simulink model "AGTF30SysDyn_PExPIn"  (R2023b)
settings: Solver=ode4  StartTime=0.0  StopTime=MWS.In.tend  FixedStep=MWS.In.Ts  RelTol=1e-3  EnableMultiTasking=on
model workspace: external: MAT-File (data not in the file)
values from neighbouring files (symbols this model uses):
  MWS = setup_initialize(MWS,startPt,SSsolverSP)    [Setup_Simulation.m]    (also in run_AGTF30e_script.m = Setup_Simulation(inputMethod,MWS.In,filename,Mdl,SSsolverSP))
undefined symbols (not defined in the file or in its folder): DiscIntNeverNeededParam
libraries: simulink x32, Lib_Solve_ModelSource_TMATS x28, Lib_EMTAT x27, Lib_Cntrl_FirstOrderSensor_TMATS x19, Lib_Cntrl_FirstOrderActuator_TMATS x2, Lib_Cntrl_LimitSelect_TMATS x2, Lib_Solve_OuterLoopIntegrator_TMATS x2, Lib_Cntrl_CorrectedSpeed_TMATS x1, Lib_Solve_IterNRSolverJC_TMATS x1, slpidlib x1
(part 6 of 8)

== system AGTF30SysDyn_PExPIn/Control System/Scheduling/Steady State EM Power - MaxMin/HP and LP Pwr Calc/Gearbox Speeds/Spool to PGB speeds ==
  note: Sun
      | Ring
      | Carrier
  note: Sun
      | Ring
      | Carrier
  N : Inport
  Constant : Constant  Value=MWS.In.Options.PGBConfig
  Demux1 : Demux  Outputs=2
  Epicyclic Gearbox Speed Calc - RC : Subsystem  mask(Epicyclic Gearbox Speed Calc - SC){rS_M=MWS.Shaft.PGB.Sun.r, rR_M=MWS.Shaft.PGB.Ring.r}
      mask prompts: rS_M "rS_M - Sun gear radius, ft"; rR_M "rR_M - Ring gear radius, ft"
      mask help: This block outputs the rotational speeds of all 4 epicyclic gearbox components (sun, ring, carrier, planets) given the speeds of the sun gear and carrier. Units are consistent with input units.
      mask init:
      | rP_I = 0.5*(rR_M-rS_M);
  Epicyclic Gearbox Speed Calc - RC1 : Subsystem  mask(Epicyclic Gearbox Speed Calc - SC){rS_M=MWS.Shaft.PGB.Sun.r, rR_M=MWS.Shaft.PGB.Ring.r}
      mask prompts: rS_M "rS_M - Sun gear radius, ft"; rR_M "rR_M - Ring gear radius, ft"
      mask help: This block outputs the rotational speeds of all 4 epicyclic gearbox components (sun, ring, carrier, planets) given the speeds of the sun gear and carrier. Units are consistent with input units.
      mask init:
      | rP_I = 0.5*(rR_M-rS_M);
  Epicyclic Gearbox Speed Calc - SC : Subsystem  mask(Epicyclic Gearbox Speed Calc - SC){rS_M=MWS.Shaft.PGB.Sun.r, rR_M=MWS.Shaft.PGB.Ring.r}
      mask prompts: rS_M "rS_M - Sun gear radius, ft"; rR_M "rR_M - Ring gear radius, ft"
      mask help: This block outputs the rotational speeds of all 4 epicyclic gearbox components (sun, ring, carrier, planets) given the speeds of the sun gear and carrier. Units are consistent with input units.
      mask init:
      | rP_I = 0.5*(rR_M-rS_M);
  Epicyclic Gearbox Speed Calc - SC1 : Subsystem  mask(Epicyclic Gearbox Speed Calc - SC){rS_M=MWS.Shaft.PGB.Sun.r, rR_M=MWS.Shaft.PGB.Ring.r}
      mask prompts: rS_M "rS_M - Sun gear radius, ft"; rR_M "rR_M - Ring gear radius, ft"
      mask help: This block outputs the rotational speeds of all 4 epicyclic gearbox components (sun, ring, carrier, planets) given the speeds of the sun gear and carrier. Units are consistent with input units.
      mask init:
      | rP_I = 0.5*(rR_M-rS_M);
  Epicyclic Gearbox Speed Calc - SR : Subsystem  mask(Epicyclic Gearbox Speed Calc - SR){rS_M=MWS.Shaft.PGB.Sun.r, rR_M=MWS.Shaft.PGB.Ring.r}
      mask prompts: rS_M "rS_M - Radius of the sun gear, ft"; rR_M "rR_M - Radius of the ring gear, ft"
      mask help: This block outputs the rotational speeds of all 4 epicyclic gearbox components (sun, ring, carrier, planets) given the speeds of the sun gear and ring gear. Units are consistent with input units.
      mask init:
      | rP_I = 0.5*(rR_M-rS_M);
  Epicyclic Gearbox Speed Calc - SR1 : Subsystem  mask(Epicyclic Gearbox Speed Calc - SR){rS_M=MWS.Shaft.PGB.Sun.r, rR_M=MWS.Shaft.PGB.Ring.r}
      mask prompts: rS_M "rS_M - Radius of the sun gear, ft"; rR_M "rR_M - Radius of the ring gear, ft"
      mask help: This block outputs the rotational speeds of all 4 epicyclic gearbox components (sun, ring, carrier, planets) given the speeds of the sun gear and ring gear. Units are consistent with input units.
      mask init:
      | rP_I = 0.5*(rR_M-rS_M);
  Gain1 : Gain  Gain=MWS.Shaft.PGB.Sun.GR_gb %GR = Ngb/Nint
  Gain19 : Gain  Gain=MWS.Shaft.PGB.Ring.GR_gb %GR = Ngb/Nint
  Gain2 : Gain  Gain=MWS.Shaft.PGB.Sun.GR_int %GR = Nint/Ncomp
  Gain20 : Gain  Gain=MWS.Shaft.PGB.Carrier.GR_int %GR = Nint/Ncomp
  Gain21 : Gain  Gain=MWS.Shaft.PGB.Carrier.GR_gb %GR = Ngb/Nint
  Gain22 : Gain  Gain=MWS.Shaft.PGB.Ring.GR_int %GR = Nint/Ncomp
  Gain23 : Gain  Gain=MWS.Shaft.PGB.Sun.GR_gb %GR = Ngb/Nint
  Gain24 : Gain  Gain=MWS.Shaft.PGB.Ring.GR_gb %GR = Ngb/Nint
  Gain25 : Gain  Gain=MWS.Shaft.PGB.Sun.GR_int %GR = Nint/Ncomp
  Gain26 : Gain  Gain=MWS.Shaft.PGB.Carrier.GR_int %GR = Nint/Ncomp
  Gain27 : Gain  Gain=MWS.Shaft.PGB.Carrier.GR_gb %GR = Ngb/Nint
  Gain28 : Gain  Gain=MWS.Shaft.PGB.Ring.GR_int %GR = Nint/Ncomp
  Multiport Switch2 : MultiPortSwitch  Inputs=6  SaturateOnIntegerOverflow=off  InputSameDT=off
  NPGB : Outport
  wires:
  Demux1/1 -> Gain20/1, Gain22/1, Gain2/1  "N2"
  Gain27/1 -> [NC_HP]
  Epicyclic Gearbox Speed Calc - RC1/1(N) -> Multiport Switch2/7
  Epicyclic Gearbox Speed Calc - SR1/1(N) -> Multiport Switch2/4
  Gain22/1 -> Gain19/1
  [NS_LP] -> Epicyclic Gearbox Speed Calc - SR1/1(NS)
  [NR_LP] -> Epicyclic Gearbox Speed Calc - RC1/1(NR)
  N/1 -> Demux1/1
  Gain20/1 -> Gain21/1
  Gain28/1 -> Gain24/1
  [NC_LP] -> Epicyclic Gearbox Speed Calc - SC/2(NC)
  Gain2/1 -> Gain1/1
  [NS_HP] -> Epicyclic Gearbox Speed Calc - SC/1(NS)
  Multiport Switch2/1 -> NPGB/1
  [NR_LP] -> Epicyclic Gearbox Speed Calc - SR/2(NR)
  Gain24/1 -> [NR_HP]
  [NR_HP] -> Epicyclic Gearbox Speed Calc - RC/1(NR)
  Demux1/2 -> Gain26/1, Gain28/1, Gain25/1  "N3"
  Gain26/1 -> Gain27/1
  Gain25/1 -> Gain23/1
  Gain1/1 -> [NS_LP]
  Epicyclic Gearbox Speed Calc - SC/1(N) -> Multiport Switch2/3
  [NS_HP] -> Epicyclic Gearbox Speed Calc - SR/1(NS)
  Gain19/1 -> [NR_LP]
  Gain21/1 -> [NC_LP]
  Gain23/1 -> [NS_HP]
  Epicyclic Gearbox Speed Calc - SR/1(N) -> Multiport Switch2/2
  [NC_HP] -> Epicyclic Gearbox Speed Calc - SC1/2(NC)
  [NC_HP] -> Epicyclic Gearbox Speed Calc - RC1/2(NC)
  [NS_LP] -> Epicyclic Gearbox Speed Calc - SC1/1(NS)
  Epicyclic Gearbox Speed Calc - RC/1(N) -> Multiport Switch2/5
  Constant/1 -> Multiport Switch2/1
  [NR_HP] -> Epicyclic Gearbox Speed Calc - SR1/2(NR)
  [NC_LP] -> Epicyclic Gearbox Speed Calc - RC/2(NC)
  Epicyclic Gearbox Speed Calc - SC1/1(N) -> Multiport Switch2/6

== system AGTF30SysDyn_PExPIn/EngineSystem/Power System/Electrical Power System/EM Variant Subsystem/Scalar DEM Subsystem/PCabqPEM Calc ==
  CablePwr : Inport
  EMPwr : Inport  Port=2
  Divide1 : Product  Inputs=*/
  Memory : Memory  InitialCondition=1
  Saturation : Saturate  UpperLimit=1/0.2  LowerLimit=0.2
  Switch : Switch  Criteria=u2 > Threshold  SaturateOnIntegerOverflow=off  InputSameDT=off
  W to hp2 : Gain  Gain=1/745.7
  Zero Check2 : Subsystem
  PCabqPEM : Outport
  wires:
  Memory/1 -> Switch/1
  W to hp2/1 -> Divide1/1
  Zero Check2/2(Check) -> Switch/2
  Saturation/1 -> PCabqPEM/1, Memory/1
  CablePwr/1 -> W to hp2/1
  Zero Check2/1(EMPwrNZ) -> Divide1/2
  EMPwr/1 -> Zero Check2/1(EMPwr)
  Divide1/1 -> Switch/3
  Switch/1 -> Saturation/1

== system AGTF30SysDyn_PExPIn/EngineSystem/Power System/Electrical Power System/EM Variant Subsystem/Scalar DEM Subsystem/PCabqPEM Calc1 ==
  CablePwr : Inport
  EMPwr : Inport  Port=2
  Divide1 : Product  Inputs=*/
  Memory : Memory  InitialCondition=1
  Saturation : Saturate  UpperLimit=1/0.2  LowerLimit=0.2
  Switch : Switch  Criteria=u2 > Threshold  SaturateOnIntegerOverflow=off  InputSameDT=off
  W to hp2 : Gain  Gain=1/745.7
  Zero Check2 : Subsystem
  PCabqPEM : Outport
  wires:
  Switch/1 -> Saturation/1
  Divide1/1 -> Switch/3
  EMPwr/1 -> Zero Check2/1(EMPwr)
  Zero Check2/1(EMPwrNZ) -> Divide1/2
  CablePwr/1 -> W to hp2/1
  Saturation/1 -> Memory/1, PCabqPEM/1
  Zero Check2/2(Check) -> Switch/2
  W to hp2/1 -> Divide1/1
  Memory/1 -> Switch/1

== system AGTF30SysDyn_PExPIn/EngineSystem/Power System/Electrical Power System/EM Variant Subsystem/Scalar PGB EM Subsystem/PCabqPEM Calc ==
  CablePwr : Inport
  EMPwr : Inport  Port=2
  Divide1 : Product  Inputs=*/
  Memory : Memory  InitialCondition=1
  Saturation : Saturate  UpperLimit=1/0.2  LowerLimit=0.2
  Switch : Switch  Criteria=u2 > Threshold  SaturateOnIntegerOverflow=off  InputSameDT=off
  W to hp2 : Gain  Gain=1/745.7
  Zero Check2 : Subsystem
  PCabqPEM : Outport
  wires:
  Memory/1 -> Switch/1
  W to hp2/1 -> Divide1/1
  Zero Check2/2(Check) -> Switch/2
  Saturation/1 -> PCabqPEM/1, Memory/1
  CablePwr/1 -> W to hp2/1
  Zero Check2/1(EMPwrNZ) -> Divide1/2
  EMPwr/1 -> Zero Check2/1(EMPwr)
  Switch/1 -> Saturation/1
  Divide1/1 -> Switch/3

== system AGTF30SysDyn_PExPIn/EngineSystem/Power System/Electrical Power System/EM Variant Subsystem/Scalar PGB EM Subsystem/PCabqPEM Calc1 ==
  CablePwr : Inport
  EMPwr : Inport  Port=2
  Divide1 : Product  Inputs=*/
  Memory : Memory  InitialCondition=1
  Saturation : Saturate  UpperLimit=1/0.2  LowerLimit=0.2
  Switch : Switch  Criteria=u2 > Threshold  SaturateOnIntegerOverflow=off  InputSameDT=off
  W to hp2 : Gain  Gain=1/745.7
  Zero Check2 : Subsystem
  PCabqPEM : Outport
  wires:
  Memory/1 -> Switch/1
  W to hp2/1 -> Divide1/1
  Zero Check2/2(Check) -> Switch/2
  Saturation/1 -> PCabqPEM/1, Memory/1
  CablePwr/1 -> W to hp2/1
  Zero Check2/1(EMPwrNZ) -> Divide1/2
  EMPwr/1 -> Zero Check2/1(EMPwr)
  Divide1/1 -> Switch/3
  Switch/1 -> Saturation/1

== system AGTF30SysDyn_PExPIn/EngineSystem/Power System/Electrical Power System/EM Variant Subsystem/Scalar PGB EM Subsystem/PCabqPEM Calc2 ==
  CablePwr : Inport
  EMPwr : Inport  Port=2
  Divide1 : Product  Inputs=*/
  Memory : Memory  InitialCondition=1
  Saturation : Saturate  UpperLimit=1/0.2  LowerLimit=0.2
  Switch : Switch  Criteria=u2 > Threshold  SaturateOnIntegerOverflow=off  InputSameDT=off
  W to hp2 : Gain  Gain=1/745.7
  Zero Check2 : Subsystem
  PCabqPEM : Outport
  wires:
  Memory/1 -> Switch/1
  W to hp2/1 -> Divide1/1
  Zero Check2/2(Check) -> Switch/2
  Saturation/1 -> PCabqPEM/1, Memory/1
  CablePwr/1 -> W to hp2/1
  Zero Check2/1(EMPwrNZ) -> Divide1/2
  EMPwr/1 -> Zero Check2/1(EMPwr)
  Divide1/1 -> Switch/3
  Switch/1 -> Saturation/1

== system AGTF30SysDyn_PExPIn/EngineSystem/Power System/Electrical Power System/EM Variant Subsystem/Scalar PGB EM Subsystem/PCabqPEM Calc3 ==
  CablePwr : Inport
  EMPwr : Inport  Port=2
  Divide1 : Product  Inputs=*/
  Memory : Memory  InitialCondition=1
  Saturation : Saturate  UpperLimit=1/0.2  LowerLimit=0.2
  Switch : Switch  Criteria=u2 > Threshold  SaturateOnIntegerOverflow=off  InputSameDT=off
  W to hp2 : Gain  Gain=1/745.7
  Zero Check2 : Subsystem
  PCabqPEM : Outport
  wires:
  Memory/1 -> Switch/1
  W to hp2/1 -> Divide1/1
  Zero Check2/2(Check) -> Switch/2
  Saturation/1 -> PCabqPEM/1, Memory/1
  CablePwr/1 -> W to hp2/1
  Zero Check2/1(EMPwrNZ) -> Divide1/2
  EMPwr/1 -> Zero Check2/1(EMPwr)
  Divide1/1 -> Switch/3
  Switch/1 -> Saturation/1

== system AGTF30SysDyn_PExPIn/EngineSystem/Power System/Electrical Power System/Energy Storage Subsystem/DCDC Variant Subsystem/DCDC Regulator Subsystem ==
  V_ESD [V] : Inport
  I_Bus [A] : Inport  Port=2
  Constant : Constant  Value=MWS.EPS.DCDC.Vset
  Constant129 : Constant  Value=0
  Constant39 : Constant  Value=0
  DC-DC Converter (Efficiency Map) (Regulate Output Voltage) : Lib_EMTAT/Components/Power Flow/DC-DC Converter (Efficiency Map) (Regulate Output Voltage)  X_Vin_VoltageVec_M=MWS.EPS.DCDC.Vvec  Y_Iout_CurrentVec_M=MWS.EPS.DCDC.Ivec  T_C_EffArray_M=MWS.EPS.DCDC.Eff  FM=0
      settings: SourceProductName=EMTAT
      settings: AttributesFormatString=|
      | DC-DC Converter
      | (Efficiency Map)
      | (Regulate Output Voltage)
  Electrical Bus : Lib_EMTAT/Components/Power Flow/Electrical Bus  C=MWS.EPS.Bus.C  Nb=1
      settings: AttributesFormatString=Electrical Bus  SourceProductName=EMTAT
  Gain : Gain  Gain=-1
  Gain1 : Gain  Gain=-1
  Integrator : Integrator  InitialCondition=MWS.EPS.Bus.Vout_IC
  Mux : Mux  Inputs=2
  PID Controller : slpidlib/PID Controller  Controller=PID  Form=Parallel  TimeDomain=Continuous-time  UseExternalTs=off  SampleTime=-1  IntegratorMethod=Forward Euler  FilterMethod=Forward Euler  ControllerParametersSource=internal  P=MWS.EPS.DCDC.PID.kp  I=MWS.EPS.DCDC.PID.ki  UseKiTs=off  D=MWS.EPS.DCDC.PID.kd  N=100  UseFilter=on  TunerSelectOption=Frequency Response Based  InitialConditionSource=internal  InitialConditionForIntegrator=0  InitialConditionForFilter=0  DifferentiatorICPrevScaledInput=0  ExternalReset=none  TrackingMode=off  Kt=1  LimitOutput=off  SatLimitsSource=internal  UpperSaturationLimit=inf  LowerSaturationLimit=-inf  LinearizeAsGain=on  AntiWindupMode=none  Kb=1  LimitIntegrator=off  UpperIntegratorSaturationLimit=inf  LowerIntegratorSaturationLimit=-inf  POutMin=[]  POutMax=[]  IOutMin=[]  IOutMax=[]  DOutMin=[]  DOutMax=[]  NOutMin=[]  NOutMax=[]  SumOutMin=[]  SumOutMax=[]  SaturationOutMin=[]  SaturationOutMax=[]  PParamMin=[]  PParamMax=[]  IParamMin=[]  IParamMax=[]  DParamMin=[]  DParamMax=[]  NParamMin=[]  NParamMax=[]  KbParamMin=[]  KbParamMax=[]  KtParamMin=[]  KtParamMax=[]  KbOutMin=[]  KbOutMax=[]  KtOutMin=[]  KtOutMax=[]  IntegratorOutMin=[]  IntegratorOutMax=[]  FilterOutMin=[]  FilterOutMax=[]  SumI1OutMin=[]  SumI1OutMax=[]  SumI2OutMin=[]  SumI2OutMax=[]  SumI3OutMin=[]  SumI3OutMax=[]  SumI4OutMin=[]  SumI4OutMax=[]  SumDOutMin=[]  SumDOutMax=[]  DifferentiatorOutMin=[]  DifferentiatorOutMax=[]  FilterDiffOutCoefMin=[]  FilterDiffOutCoefMax=[]  ReciprocalOutMin=[]  ReciprocalOutMax=[]  SumDenOutMin=[]  SumDenOutMax=[]  SumNumOutMin=[]  SumNumOutMax=[]  DivideOutMin=[]  DivideOutMax=[]  UdiffTsProdOutMin=[]  UdiffTsProdOutMax=[]  NTsProdOutMin=[]  NTsProdOutMax=[]  UintegralTsProdOutMin=[]  UintegralTsProdOutMax=[]  UngainTsProdOutMin=[]  UngainTsProdOutMax=[]  ClampingZeroOutDataTypeStr=Inherit: Inherit via back propagation  ClampingZeroOutMin=[]  ClampingZeroOutMax=[]  FilterDenConstantOutDataTypeStr=Inherit: Inherit via back propagation  FilterDenConstantOutMin=[]  FilterDenConstantOutMax=[]  PCopyOutDataTypeStr=Inherit: Inherit via back propagation  PCopyOutMin=[]  PCopyOutMax=[]  NCopyOutDataTypeStr=Inherit: Inherit via back propagation  NCopyOutMin=[]  NCopyOutMax=[]  IntegratorContinuousStateAttributes=''  IntegratorStateMustResolveToSignalObject=off  IntegratorRTWStateStorageClass=Auto  FilterContinuousStateAttributes=''  FilterStateMustResolveToSignalObject=off  FilterRTWStateStorageClass=Auto  ParallelPVariant=InternalParameters  IdealPVariant=Disabled  IVariant=InternalParameters  DVariant=InternalParameters  IntegratorVariant=Continuous  SatVariant=Disabled  AWVariant=Passthrough  PCopyVariant=Disabled  TRVariant=Disabled  FdbkBlocksVariant=Forward  IdealPFdbkVariant=Disabled  SatFdbkVariant=Disabled  DerivativeFilterVariant=ContFilter  NVariant=InternalParameters  NCopyVariant=Disabled  FilterICVariant=InternalICsFilter  IntegratorICVariant=InternalICs  ExternalResetVariant=Disabled  TRSumVariant=Passthrough  SumFdbkVariant=Disabled  SumVariant=Sum_PID  TsampFilterVariant=InternalTs  TsampNgainVariant=Passthrough  TsampIntegralVariant=Disabled_SignalSpec  ExternalSaturationOutDataTypeStr=Inherit: Same as second input
  Sum : Sum  Inputs=-+
  Sum of Elements : Sum  Inputs=+
  Terminator46 : Terminator
  Vo [V] : Outport
  Io [A] : Outport  Port=2
  Outputs : Outport  Port=3
  wires:
  Constant39/1 -> DC-DC Converter (Efficiency Map) (Regulate Output Voltage)/4
  I_Bus [A]/1 -> Mux/2
  Constant129/1 -> DC-DC Converter (Efficiency Map) (Regulate Output Voltage)/5
  DC-DC Converter (Efficiency Map) (Regulate Output Voltage)/2 -> Terminator46/1
  DC-DC Converter (Efficiency Map) (Regulate Output Voltage)/1 -> Outputs/1
  Electrical Bus/2 -> Integrator/1
  Integrator/1 -> Electrical Bus/2
  Electrical Bus/1 -> Vo [V]/1, DC-DC Converter (Efficiency Map) (Regulate Output Voltage)/2, Sum/1
  DC-DC Converter (Efficiency Map) (Regulate Output Voltage)/3 -> Gain/1
  Constant/1 -> Sum/2
  PID Controller/1 -> DC-DC Converter (Efficiency Map) (Regulate Output Voltage)/3
  Sum/1 -> PID Controller/1
  Gain/1 -> Mux/1
  Sum of Elements/1 -> Gain1/1
  Gain1/1 -> Electrical Bus/1
  V_ESD [V]/1 -> DC-DC Converter (Efficiency Map) (Regulate Output Voltage)/1
  DC-DC Converter (Efficiency Map) (Regulate Output Voltage)/4 -> Io [A]/1
  Mux/1 -> Sum of Elements/1

== system AGTF30SysDyn_PExPIn/EngineSystem/Power System/Electrical Power System/Energy Storage Subsystem/DCDC Variant Subsystem/DCDC Set Point Subsystem ==
  V_ESD [V] : Inport
  I_Bus [A] : Inport  Port=2
  Constant : Constant  Value=MWS.EPS.DCDC.Vset
  Constant129 : Constant  Value=0
  Constant39 : Constant  Value=0
  DC-DC Converter (Efficiency Map) (Regulate Output Voltage) : Lib_EMTAT/Components/Power Flow/DC-DC Converter (Efficiency Map) (Regulate Output Voltage)  X_Vin_VoltageVec_M=MWS.EPS.DCDC.Vvec  Y_Iout_CurrentVec_M=MWS.EPS.DCDC.Ivec  T_C_EffArray_M=MWS.EPS.DCDC.Eff  FM=0
      settings: SourceProductName=EMTAT
      settings: AttributesFormatString=|
      | DC-DC Converter
      | (Efficiency Map)
      | (Regulate Output Voltage)
  Terminator46 : Terminator
  Unit Delay1 : UnitDelay  SampleTime=-1  HasFrameUpgradeWarning=on
  Vo [V] : Outport
  Io [A] : Outport  Port=2
  Outputs : Outport  Port=3
  wires:
  Constant39/1 -> DC-DC Converter (Efficiency Map) (Regulate Output Voltage)/4
  DC-DC Converter (Efficiency Map) (Regulate Output Voltage)/2 -> Outputs/1
  Constant/1 -> DC-DC Converter (Efficiency Map) (Regulate Output Voltage)/1
  V_ESD [V]/1 -> DC-DC Converter (Efficiency Map) (Regulate Output Voltage)/2
  Constant129/1 -> DC-DC Converter (Efficiency Map) (Regulate Output Voltage)/5
  I_Bus [A]/1 -> DC-DC Converter (Efficiency Map) (Regulate Output Voltage)/3
  DC-DC Converter (Efficiency Map) (Regulate Output Voltage)/4 -> Unit Delay1/1
  DC-DC Converter (Efficiency Map) (Regulate Output Voltage)/3 -> Terminator46/1
  DC-DC Converter (Efficiency Map) (Regulate Output Voltage)/1 -> Vo [V]/1
  Unit Delay1/1 -> Io [A]/1

== system AGTF30SysDyn_PExPIn/EngineSystem/Power System/Electrical Power System/Energy Storage Subsystem/ESD Variant Subsystem/ESD Battery Subsystem ==
  I [A] : Inport
  Battery : Lib_EMTAT/Components/Power Flow/Battery  ESR=MWS.EPS.Batt.ESR  Vcharge_vec=MWS.EPS.Batt.VCC  Vdischarge_vec=MWS.EPS.Batt.VDC  It_vec=MWS.EPS.Batt.DoD
      settings: AttributesFormatString=Battery  SourceProductName=EMTAT
  Bus Selector : BusSelector  OutputSignals=SoC; %
  Integrator : Integrator  InitialCondition=MWS.EPS.Batt.DoD_IC
  Terminator46 : Terminator
  Vo [V] : Outport
  SoC [%] : Outport  Port=2
  wires:
  Bus Selector/1 -> SoC [%]/1  "<SoC; %>"
  Battery/2 -> Bus Selector/1
  I [A]/1 -> Battery/1
  Battery/4 -> Integrator/1
  Integrator/1 -> Battery/2
  Battery/3 -> Terminator46/1
  Battery/1 -> Vo [V]/1

== system AGTF30SysDyn_PExPIn/EngineSystem/Power System/Electrical Power System/Energy Storage Subsystem/ESD Variant Subsystem/ESD Supercapacitor Subsystem ==
  I [A] : Inport
  Bus Selector : BusSelector  OutputSignals=SOC; %
  Integrator : Integrator  InitialCondition=MWS.EPS.SC.Vout_IC
  Supercapacitor : Lib_EMTAT/Components/Power Flow/Supercapacitor  C=MWS.EPS.SC.C  ESR=MWS.EPS.SC.ESR  TSE=MWS.EPS.SC.TSE  BlkNm=double(gcb)
      settings: AttributesFormatString=Supercapacitor  SourceProductName=EMTAT
  Terminator46 : Terminator
  Unit Delay : UnitDelay  InitialCondition=MWS.EPS.SC.Iout_IC  SampleTime=-1  HasFrameUpgradeWarning=on
  Vo [V] : Outport
  SoC [%] : Outport  Port=2
  wires:
  Integrator/1 -> Supercapacitor/2
  Supercapacitor/4 -> Integrator/1
  Supercapacitor/3 -> Terminator46/1
  Supercapacitor/1 -> Vo [V]/1  "Vout (Supercapacitor) [V]"
  Supercapacitor/5 -> Unit Delay/1
  Unit Delay/1 -> Supercapacitor/3
  I [A]/1 -> Supercapacitor/1
  Supercapacitor/2 -> Bus Selector/1
  Bus Selector/1 -> SoC [%]/1  "<SOC; %>"

== system AGTF30SysDyn_PExPIn/Control System/Electric Machine Controllers/EM Controllers/PGB EM Control/VEATE EM Controllers/Base Power/Base Power - Boost and PEx ==
  note: 1: HP-Sun, LP-Ring, Coupling-Carrier
      | 2: HP-Sun, LP-Carrier, Coupling-Ring
      | 3: HP-Ring, LP-Sun, Coupling-Carrier
      | 4: HP-Ring, LP-Carrier, Coupling-Sun
      | 5: HP-Carrier, LP-Sun, Coupling-Ring
      | 6: HP-Carrier, LP-Ring, Coupling-Sun
  note: PLANETARY GEARBOX EFFECT ON POWER TRANSFER
  PwrL_Base : Inport
  PwrH_Base : Inport  Port=2
  NS : Inport  Port=3
  NR : Inport  Port=4
  NC : Inport  Port=5
  Boost PEx - HC LR CS : Subsystem
  Boost PEx - HC LS CR : Subsystem
  Boost PEx - HR LC CS : Subsystem
  Boost PEx - HR LS CC : Subsystem
  Boost PEx - HS LC CR : Subsystem
  Boost PEx - HS LR CC : Subsystem
  CTrqCR : Constant  Value=MWS.Shaft.PGB.TrqCoeff.CTrqCR
  CTrqCS : Constant  Value=MWS.Shaft.PGB.TrqCoeff.CTrqCS
  CTrqRC : Constant  Value=MWS.Shaft.PGB.TrqCoeff.CTrqRC
  CTrqRS : Constant  Value=MWS.Shaft.PGB.TrqCoeff.CTrqRS
  CTrqSC : Constant  Value=MWS.Shaft.PGB.TrqCoeff.CTrqSC
  CTrqSR : Constant  Value=MWS.Shaft.PGB.TrqCoeff.CTrqSR
  Constant1 : Constant  Value=MWS.In.Options.PGBConfig
  Constant2 : Constant  Value=MWS.In.Options.PGBConfig
  Constant3 : Constant  Value=MWS.In.Options.PGBConfig
  Divide{4..7,12..13} (6 alike) : Product  Inputs=**/
  Multiport Switch1 : MultiPortSwitch  Inputs=6  SaturateOnIntegerOverflow=off  InputSameDT=off
  Multiport Switch4 : MultiPortSwitch  Inputs=6  SaturateOnIntegerOverflow=off  InputSameDT=off
  Multiport Switch8 : MultiPortSwitch  Inputs=6  SaturateOnIntegerOverflow=off  InputSameDT=off
  Mux{1..6} (6 alike) : Mux
  Pem : Outport
  wires:
  Boost PEx - HC LS CR/1(PemS_Base) -> Mux5/1
  Boost PEx - HC LR CS/1(PemS_Base) -> Mux6/1
  Boost PEx - HC LS CR/4(PemP_Base) -> Mux5/4
  Boost PEx - HC LR CS/2(PemR_Base) -> Mux6/2
  Boost PEx - HC LR CS/3(PemC_Base) -> Mux6/3
  Mux4/1 -> [Pem_HRLCCS]
  Mux6/1 -> [Pem_HCLRCS]
  Boost PEx - HC LS CR/3(PemC_Base) -> Mux5/3
  Boost PEx - HS LC CR/3(PemC_Base) -> Mux2/3
  Boost PEx - HS LR CC/2(PemR_Base) -> Mux1/2
  Boost PEx - HR LS CC/1(PemS_Base) -> Mux3/1
  Mux1/1 -> [Pem_HSLRCC]
  Boost PEx - HS LR CC/4(PemP_Base) -> Mux1/4
  Constant1/1 -> Multiport Switch4/1
  [Pem_HSLCCR] -> Multiport Switch4/3
  Boost PEx - HC LR CS/4(PemP_Base) -> Mux6/4
  [Pem_HRLCCS] -> Multiport Switch4/5
  Boost PEx - HS LC CR/1(PemS_Base) -> Mux2/1
  Boost PEx - HC LS CR/2(PemR_Base) -> Mux5/2
  Boost PEx - HS LC CR/2(PemR_Base) -> Mux2/2
  Boost PEx - HS LC CR/4(PemP_Base) -> Mux2/4
  Boost PEx - HR LS CC/2(PemR_Base) -> Mux3/2
  Mux5/1 -> [Pem_HCLSCR]
  Boost PEx - HR LC CS/2(PemR_Base) -> Mux4/2
  Boost PEx - HR LS CC/4(PemP_Base) -> Mux3/4
  [Pem_HCLSCR] -> Multiport Switch4/6
  Boost PEx - HR LS CC/3(PemC_Base) -> Mux3/3
  Boost PEx - HR LC CS/3(PemC_Base) -> Mux4/3
  [Pem_HSLRCC] -> Multiport Switch4/2
  Mux3/1 -> [Pem_HRLSCC]
  Boost PEx - HR LC CS/4(PemP_Base) -> Mux4/4
  Boost PEx - HR LC CS/1(PemS_Base) -> Mux4/1
  Boost PEx - HS LR CC/3(PemC_Base) -> Mux1/3
  Boost PEx - HS LR CC/1(PemS_Base) -> Mux1/1
  [Pem_HCLRCS] -> Multiport Switch4/7
  [Pem_HRLSCC] -> Multiport Switch4/4
  Multiport Switch4/1 -> Pem/1
  Mux2/1 -> [Pem_HSLCCR]
  [K_PXeffRC] -> Multiport Switch8/4
  [K_PXeffCR] -> Multiport Switch8/6
  [K_PXeffSC] -> Multiport Switch8/2
  [K_PXeffCR] -> Multiport Switch1/3
  Multiport Switch1/1 -> [K_PXeffL]
  [K_PXeffCS] -> Multiport Switch1/5
  [K_PXeffSC] -> Multiport Switch1/4
  Constant3/1 -> Multiport Switch1/1
  [K_PXeffCS] -> Multiport Switch8/7
  CTrqRC/1 -> Divide12/1
  Divide7/1 -> [K_PXeffRS]
  [NC] -> Divide6/3
  [NS] -> Divide5/2
  [NS] -> Divide13/3
  Divide5/1 -> [K_PXeffSR]
  Divide12/1 -> [K_PXeffRC]
  CTrqSR/1 -> Divide5/1
  Multiport Switch8/1 -> [K_PXeffH]
  [NS] -> Divide6/2
  [NR] -> Divide7/2
  Divide13/1 -> [K_PXeffCS]
  [K_PXeffRS] -> Multiport Switch1/7
  CTrqCS/1 -> Divide13/1
  [NR] -> Divide5/3
  [K_PXeffRC] -> Multiport Switch1/2
  [NR] -> Divide12/2
  Constant2/1 -> Multiport Switch8/1
  [NR] -> Divide4/3
  CTrqCR/1 -> Divide4/1
  CTrqRS/1 -> Divide7/1
  [NC] -> Divide13/2
  CTrqSC/1 -> Divide6/1
  Divide6/1 -> [K_PXeffSC]
  [K_PXeffSR] -> Multiport Switch8/3
  Divide4/1 -> [K_PXeffCR]
  [NC] -> Divide4/2
  [NC] -> Divide12/3
  [K_PXeffSR] -> Multiport Switch1/6
  [NS] -> Divide7/3
  [K_PXeffRS] -> Multiport Switch8/5
  PwrL_Base/1 -> [PwrL_Base]
  PwrH_Base/1 -> [PwrH_Base]
  NS/1 -> [NS]
  NR/1 -> [NR]
  NC/1 -> [NC]
  [PwrH_Base] -> Boost PEx - HS LR CC/2(PwrH_Base), Boost PEx - HC LR CS/2(PwrH_Base), Boost PEx - HC LS CR/2(PwrH_Base), Boost PEx - HR LC CS/2(PwrH_Base), Boost PEx - HR LS CC/2(PwrH_Base), Boost PEx - HS LC CR/2(PwrH_Base)
  [PwrL_Base] -> Boost PEx - HS LR CC/1(PwrL_Base), Boost PEx - HC LR CS/1(PwrL_Base), Boost PEx - HC LS CR/1(PwrL_Base), Boost PEx - HR LC CS/1(PwrL_Base), Boost PEx - HR LS CC/1(PwrL_Base), Boost PEx - HS LC CR/1(PwrL_Base)
  [K_PXeffH] -> Boost PEx - HS LR CC/4(K_PXeffH), Boost PEx - HC LR CS/4(K_PXeffH), Boost PEx - HC LS CR/4(K_PXeffH), Boost PEx - HR LC CS/4(K_PXeffH), Boost PEx - HR LS CC/4(K_PXeffH), Boost PEx - HS LC CR/4(K_PXeffH)
  [K_PXeffL] -> Boost PEx - HS LR CC/3(K_PXeffL), Boost PEx - HC LR CS/3(K_PXeffL), Boost PEx - HC LS CR/3(K_PXeffL), Boost PEx - HR LC CS/3(K_PXeffL), Boost PEx - HR LS CC/3(K_PXeffL), Boost PEx - HS LC CR/3(K_PXeffL)
  [NS] -> Boost PEx - HS LR CC/5(NS), Boost PEx - HC LR CS/5(NS), Boost PEx - HC LS CR/5(NS), Boost PEx - HR LC CS/5(NS), Boost PEx - HR LS CC/5(NS), Boost PEx - HS LC CR/5(NS)
  [NR] -> Boost PEx - HS LR CC/6(NR), Boost PEx - HC LR CS/6(NR), Boost PEx - HC LS CR/6(NR), Boost PEx - HR LC CS/6(NR), Boost PEx - HR LS CC/6(NR), Boost PEx - HS LC CR/6(NR)
  [NC] -> Boost PEx - HS LR CC/7(NC), Boost PEx - HC LR CS/7(NC), Boost PEx - HC LS CR/7(NC), Boost PEx - HR LC CS/7(NC), Boost PEx - HR LS CC/7(NC), Boost PEx - HS LC CR/7(NC)

== system AGTF30SysDyn_PExPIn/Control System/Electric Machine Controllers/EM Controllers/PGB EM Control/VEATE EM Controllers/Base Power/Base Power - Standard ==
  note: 1: HP-Sun, LP-Ring, Coupling-Carrier
      | 2: HP-Sun, LP-Carrier, Coupling-Ring
      | 3: HP-Ring, LP-Sun, Coupling-Carrier
      | 4: HP-Ring, LP-Carrier, Coupling-Sun
      | 5: HP-Carrier, LP-Sun, Coupling-Ring
      | 6: HP-Carrier, LP-Ring, Coupling-Sun
  PwrH_Base : Inport
  NS : Inport  Port=2
  NR : Inport  Port=3
  NC : Inport  Port=4
  Constant1 : Constant  Value=MWS.In.Options.PGBConfig
  Multiport Switch4 : MultiPortSwitch  Inputs=6  SaturateOnIntegerOverflow=off  InputSameDT=off
  Mux1 : Mux
  Mux2 : Mux
  Mux3 : Mux
  Standard - HC : Subsystem
  Standard - HR : Subsystem
  Standard - HS : Subsystem
  Pem : Outport
  wires:
  Multiport Switch4/1 -> Pem/1
  Standard - HS/1(PemS_Base) -> Mux1/1
  Standard - HS/3(PemC_Base) -> Mux1/3
  [Pem_HS] -> Multiport Switch4/3, Multiport Switch4/2
  Constant1/1 -> Multiport Switch4/1
  Standard - HS/4(PemP_Base) -> Mux1/4
  Mux1/1 -> [Pem_HS]
  Standard - HS/2(PemR_Base) -> Mux1/2
  PwrH_Base/1 -> Standard - HC/1(PwrH_Base), Standard - HR/1(PwrH_Base), Standard - HS/1(PwrH_Base)
  NS/1 -> Standard - HS/2(NS)
  [Pem_HR] -> Multiport Switch4/5, Multiport Switch4/4
  [Pem_HC] -> Multiport Switch4/7, Multiport Switch4/6
  Standard - HR/2(PemR_Base) -> Mux2/2
  Standard - HR/4(PemP_Base) -> Mux2/4
  Standard - HR/3(PemC_Base) -> Mux2/3
  Standard - HR/1(PemS_Base) -> Mux2/1
  Mux2/1 -> [Pem_HR]
  NR/1 -> Standard - HR/2(NR)
  Mux3/1 -> [Pem_HC]
  Standard - HC/1(PemS_Base) -> Mux3/1
  Standard - HC/3(PemC_Base) -> Mux3/3
  Standard - HC/4(PemP_Base) -> Mux3/4
  Standard - HC/2(PemR_Base) -> Mux3/2
  NC/1 -> Standard - HC/2(NS)

== system AGTF30SysDyn_PExPIn/Control System/Electric Machine Controllers/EM Controllers/PGB EM Control/VEATE EM Controllers/Base Power/Load Calc ==
  note: 1: HP-Sun, LP-Ring, Coupling-Carrier
      | 2: HP-Sun, LP-Carrier, Coupling-Ring
      | 3: HP-Ring, LP-Sun, Coupling-Carrier
      | 4: HP-Ring, LP-Carrier, Coupling-Sun
      | 5: HP-Carrier, LP-Sun, Coupling-Ring
      | 6: HP-Carrier, LP-Ring, Coupling-Sun
  PemBoost_PEx : Inport
  PExAC : Inport  Port=2
  PwrSys : Inport  Port=3
  Bus Selector1 : BusSelector  OutputSignals=Pwrs.EMSbranch
  Bus Selector2 : BusSelector  OutputSignals=Pwrs.EMRbranch
  Bus Selector3 : BusSelector  OutputSignals=Pwrs.EMCbranch
  Bus Selector4 : BusSelector  OutputSignals=Pwrs.EMPbranch
  Constant1 : Constant  Value=MWS.In.Options.PGBConfig
  Demux : Demux  Outputs=[1 1 1 1]
  Demux{1..4} (4 alike) : Demux  Outputs=[4 1]
  Divide{,1..6} (7 alike) : Product  Inputs=**
  Gain1 : Gain  Gain=MWS.Shaft.PGB.Planet.nP
  Gain{2,4..9} (7 alike) : Gain  Gain=-1
  Math Function{,1..3} (4 alike) : Math  Operator=reciprocal
  Memory{,1..3} (4 alike) : Memory  InitialCondition=1
  MinMax{,1..3} (4 alike) : MinMax
  Multiport Switch4 : MultiPortSwitch  Inputs=6  SaturateOnIntegerOverflow=off  InputSameDT=off
  Mux{,1..3} (4 alike) : Mux  Inputs=2
  Sum : Sum  Inputs=|+-
  Sum2 : Sum  Inputs=|+-
  Sum3 : Sum  Inputs=|++
  Sum4 : Sum  Inputs=+|+|+|+
  Sum5 : Sum  Inputs=+|+|+|+
  Sum6 : Sum  Inputs=|++
  Sum7 : Sum  Inputs=+|+|+|+
  Sum8 : Sum  Inputs=|+-
  Sum9 : Sum  Inputs=|++
  Terminator{,1..3} (4 alike) : Terminator
  PwrLoad : Outport
  wires:
  PemBoost_PEx/1 -> Demux/1
  Demux/4 -> Gain1/1
  Demux/1 -> [PemS]
  Demux/2 -> [PemR]
  Demux/3 -> [PemC]
  Gain1/1 -> [PemP]
  Constant1/1 -> Multiport Switch4/1
  PExAC/1 -> [PExAC]
  [PemS] -> Gain2/1
  Gain2/1 -> Sum/1
  [PExAC] -> Sum3/1, Sum/2
  [PExAC] -> Sum6/1, Sum2/2
  [PemR] -> Gain4/1
  Sum/1 -> Divide/1  "Prop PEx"
  [EffS] -> Divide/2
  Divide/1 -> Sum3/2  "Prop Load"
  [PemR] -> Gain5/1
  Gain5/1 -> Divide1/1
  [EffR] -> Divide1/2
  [EffC] -> Divide2/2
  Gain6/1 -> Divide2/1
  [PemC] -> Gain6/1
  Sum3/1 -> Sum4/1  "Sun"
  Divide1/1 -> Sum4/2, Sum7/2  "Ring"
  Divide2/1 -> Sum4/3, Sum5/3  "Carrier"
  [PemP] -> Gain7/1
  Gain7/1 -> Divide3/1
  [EffP] -> Divide3/2
  Divide3/1 -> Sum5/4, Sum7/4, Sum4/4  "Planets"
  Sum4/1 -> Multiport Switch4/2, Multiport Switch4/3  "Load"
  Gain4/1 -> Sum2/1
  [EffS] -> Divide4/2
  [PemS] -> Gain8/1
  Gain8/1 -> Divide4/1
  Divide4/1 -> Sum7/1, Sum5/1  "Sun"
  [EffR] -> Divide5/2
  Sum2/1 -> Divide5/1  "Prop PEx"
  Divide5/1 -> Sum6/2  "Prop Load"
  Sum6/1 -> Sum5/2  "Ring"
  Sum5/1 -> Multiport Switch4/5, Multiport Switch4/4  "Load"
  Divide6/1 -> Sum9/2  "Prop Load"
  Gain9/1 -> Sum8/1
  Sum8/1 -> Divide6/1  "Prop PEx"
  [PemC] -> Gain9/1
  [PExAC] -> Sum9/1, Sum8/2
  [EffC] -> Divide6/2
  Sum9/1 -> Sum7/3  "Carrier"
  Sum7/1 -> Multiport Switch4/7, Multiport Switch4/6  "Load"
  Multiport Switch4/1 -> PwrLoad/1
  PwrSys/1 -> [PwrSys]
  MinMax/1 -> Memory/1
  [PwrSys] -> Bus Selector1/1
  Math Function/1 -> Mux/2
  Bus Selector1/1 -> Demux1/1  "<EMSbranch>"
  Demux1/2 -> Mux/1, Math Function/1  "PCabqPEM"
  Demux1/1 -> Terminator/1
  Memory/1 -> [EffS]
  Mux/1 -> MinMax/1
  Mux1/1 -> MinMax1/1
  Memory1/1 -> [EffR]
  Demux2/1 -> Terminator1/1
  Demux2/2 -> Math Function1/1, Mux1/1  "PCabqPEM"
  Bus Selector2/1 -> Demux2/1  "<EMRbranch>"
  Math Function1/1 -> Mux1/2
  [PwrSys] -> Bus Selector2/1
  MinMax1/1 -> Memory1/1
  MinMax2/1 -> Memory2/1
  [PwrSys] -> Bus Selector3/1
  Math Function2/1 -> Mux2/2
  Bus Selector3/1 -> Demux3/1  "<EMCbranch>"
  Demux3/2 -> Mux2/1, Math Function2/1  "PCabqPEM"
  Demux3/1 -> Terminator2/1
  Memory2/1 -> [EffC]
  Mux2/1 -> MinMax2/1
  Mux3/1 -> MinMax3/1
  Memory3/1 -> [EffP]
  Demux4/1 -> Terminator3/1
  Demux4/2 -> Math Function3/1, Mux3/1  "PCabqPEM"
  Bus Selector4/1 -> Demux4/1  "<EMPbranch>"
  Math Function3/1 -> Mux3/2
  [PwrSys] -> Bus Selector4/1
  MinMax3/1 -> Memory3/1

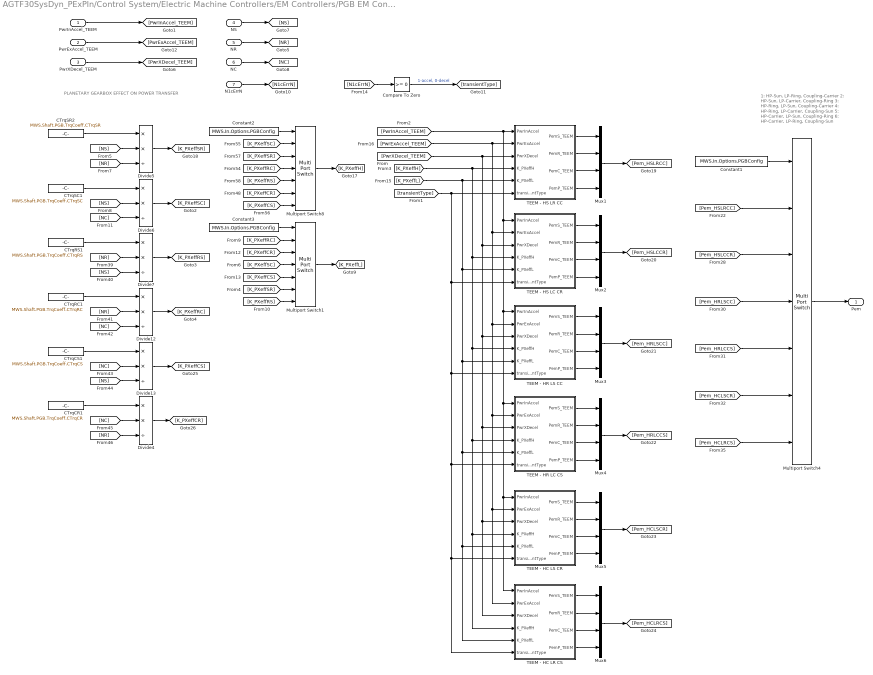
== system AGTF30SysDyn_PExPIn/Control System/Electric Machine Controllers/EM Controllers/PGB EM Control/VEATE EM Controllers/TEEM Power/TEEM Power ==
  note: 1: HP-Sun, LP-Ring, Coupling-Carrier
      | 2: HP-Sun, LP-Carrier, Coupling-Ring
      | 3: HP-Ring, LP-Sun, Coupling-Carrier
      | 4: HP-Ring, LP-Carrier, Coupling-Sun
      | 5: HP-Carrier, LP-Sun, Coupling-Ring
      | 6: HP-Carrier, LP-Ring, Coupling-Sun
  note: PLANETARY GEARBOX EFFECT ON POWER TRANSFER
  PwrInAccel_TEEM : Inport
  PwrExAccel_TEEM : Inport  Port=2
  PwrXDecel_TEEM : Inport  Port=3
  NS : Inport  Port=4
  NR : Inport  Port=5
  NC : Inport  Port=6
  N1cErrN : Inport  Port=7
  CTrqCR1 : Constant  Value=MWS.Shaft.PGB.TrqCoeff.CTrqCR
  CTrqCS1 : Constant  Value=MWS.Shaft.PGB.TrqCoeff.CTrqCS
  CTrqRC1 : Constant  Value=MWS.Shaft.PGB.TrqCoeff.CTrqRC
  CTrqRS1 : Constant  Value=MWS.Shaft.PGB.TrqCoeff.CTrqRS
  CTrqSC1 : Constant  Value=MWS.Shaft.PGB.TrqCoeff.CTrqSC
  CTrqSR2 : Constant  Value=MWS.Shaft.PGB.TrqCoeff.CTrqSR
  Compare To Zero : simulink/Logic and Bit Operations/Compare To Zero  relop=>=  OutDataTypeStr=boolean
  Constant1 : Constant  Value=MWS.In.Options.PGBConfig
  Constant2 : Constant  Value=MWS.In.Options.PGBConfig
  Constant3 : Constant  Value=MWS.In.Options.PGBConfig
  Divide{4..7,12..13} (6 alike) : Product  Inputs=**/
  Multiport Switch1 : MultiPortSwitch  Inputs=6  SaturateOnIntegerOverflow=off  InputSameDT=off
  Multiport Switch4 : MultiPortSwitch  Inputs=6  SaturateOnIntegerOverflow=off  InputSameDT=off
  Multiport Switch8 : MultiPortSwitch  Inputs=6  SaturateOnIntegerOverflow=off  InputSameDT=off
  Mux{1..6} (6 alike) : Mux
  TEEM - HC LR CS : Subsystem
  TEEM - HC LS CR : Subsystem
  TEEM - HR LC CS : Subsystem
  TEEM - HR LS CC : Subsystem
  TEEM - HS LC CR : Subsystem
  TEEM - HS LR CC : Subsystem
  Pem : Outport
  wires:
  Multiport Switch4/1 -> Pem/1
  [Pem_HRLSCC] -> Multiport Switch4/4
  [Pem_HCLRCS] -> Multiport Switch4/7
  TEEM - HS LR CC/1(PemS_TEEM) -> Mux1/1
  TEEM - HS LR CC/3(PemC_TEEM) -> Mux1/3
  TEEM - HR LC CS/1(PemS_TEEM) -> Mux4/1
  TEEM - HR LC CS/4(PemP_TEEM) -> Mux4/4
  Mux3/1 -> [Pem_HRLSCC]
  [Pem_HSLRCC] -> Multiport Switch4/2
  TEEM - HR LC CS/3(PemC_TEEM) -> Mux4/3
  TEEM - HR LS CC/3(PemC_TEEM) -> Mux3/3
  [Pem_HCLSCR] -> Multiport Switch4/6
  TEEM - HR LS CC/4(PemP_TEEM) -> Mux3/4
  TEEM - HR LC CS/2(PemR_TEEM) -> Mux4/2
  Mux5/1 -> [Pem_HCLSCR]
  TEEM - HR LS CC/2(PemR_TEEM) -> Mux3/2
  TEEM - HS LC CR/4(PemP_TEEM) -> Mux2/4
  TEEM - HS LC CR/2(PemR_TEEM) -> Mux2/2
  TEEM - HC LS CR/2(PemR_TEEM) -> Mux5/2
  TEEM - HS LC CR/1(PemS_TEEM) -> Mux2/1
  [Pem_HRLCCS] -> Multiport Switch4/5
  TEEM - HC LR CS/4(PemP_TEEM) -> Mux6/4
  [Pem_HSLCCR] -> Multiport Switch4/3
  Constant1/1 -> Multiport Switch4/1
  TEEM - HS LR CC/4(PemP_TEEM) -> Mux1/4
  Mux1/1 -> [Pem_HSLRCC]
  TEEM - HR LS CC/1(PemS_TEEM) -> Mux3/1
  TEEM - HS LR CC/2(PemR_TEEM) -> Mux1/2
  TEEM - HS LC CR/3(PemC_TEEM) -> Mux2/3
  TEEM - HC LS CR/3(PemC_TEEM) -> Mux5/3
  Mux2/1 -> [Pem_HSLCCR]
  Mux6/1 -> [Pem_HCLRCS]
  Mux4/1 -> [Pem_HRLCCS]
  TEEM - HC LR CS/3(PemC_TEEM) -> Mux6/3
  TEEM - HC LR CS/2(PemR_TEEM) -> Mux6/2
  TEEM - HC LS CR/4(PemP_TEEM) -> Mux5/4
  TEEM - HC LR CS/1(PemS_TEEM) -> Mux6/1
  TEEM - HC LS CR/1(PemS_TEEM) -> Mux5/1
  [PwrInAccel_TEEM] -> TEEM - HS LR CC/1(PwrInAccel), TEEM - HR LC CS/1(PwrInAccel), TEEM - HC LR CS/1(PwrInAccel), TEEM - HC LS CR/1(PwrInAccel), TEEM - HR LS CC/1(PwrInAccel), TEEM - HS LC CR/1(PwrInAccel)
  PwrInAccel_TEEM/1 -> [PwrInAccel_TEEM]
  PwrExAccel_TEEM/1 -> [PwrExAccel_TEEM]
  Divide7/1 -> [K_PXeffRS]
  [NR] -> Divide7/2
  CTrqSR2/1 -> Divide5/1
  [NC] -> Divide4/2
  Multiport Switch8/1 -> [K_PXeffH]
  CTrqSC1/1 -> Divide6/1
  [NS] -> Divide6/2
  [NS] -> Divide13/3
  [NS] -> Divide5/2
  Constant2/1 -> Multiport Switch8/1
  Divide12/1 -> [K_PXeffRC]
  Divide6/1 -> [K_PXeffSC]
  [NC] -> Divide13/2
  Divide5/1 -> [K_PXeffSR]
  CTrqRC1/1 -> Divide12/1
  [NC] -> Divide6/3
  [NS] -> Divide7/3
  [NC] -> Divide12/3
  [NR] -> Divide5/3
  CTrqCS1/1 -> Divide13/1
  Divide13/1 -> [K_PXeffCS]
  CTrqRS1/1 -> Divide7/1
  [NR] -> Divide4/3
  [NR] -> Divide12/2
  CTrqCR1/1 -> Divide4/1
  Divide4/1 -> [K_PXeffCR]
  [K_PXeffSR] -> Multiport Switch8/3
  [K_PXeffSC] -> Multiport Switch8/2
  [K_PXeffRC] -> Multiport Switch8/4
  [K_PXeffRS] -> Multiport Switch8/5
  [K_PXeffCS] -> Multiport Switch8/7
  [K_PXeffCR] -> Multiport Switch8/6
  PwrXDecel_TEEM/1 -> [PwrXDecel_TEEM]
  NR/1 -> [NR]
  NS/1 -> [NS]
  NC/1 -> [NC]
  N1cErrN/1 -> [N1cErrN]
  [N1cErrN] -> Compare To Zero/1
  Compare To Zero/1 -> [transientType]  "1-accel, 0-decel"
  [transientType] -> TEEM - HS LR CC/6(transientType), TEEM - HC LR CS/6(transientType), TEEM - HC LS CR/6(transientType), TEEM - HR LC CS/6(transientType), TEEM - HR LS CC/6(transientType), TEEM - HS LC CR/6(transientType)
  [K_PXeffH] -> TEEM - HS LR CC/4(K_PXeffH), TEEM - HC LR CS/4(K_PXeffH), TEEM - HC LS CR/4(K_PXeffH), TEEM - HR LC CS/4(K_PXeffH), TEEM - HR LS CC/4(K_PXeffH), TEEM - HS LC CR/4(K_PXeffH)
  [PwrXDecel_TEEM] -> TEEM - HS LR CC/3(PwrXDecel), TEEM - HC LR CS/3(PwrXDecel), TEEM - HC LS CR/3(PwrXDecel), TEEM - HR LC CS/3(PwrXDecel), TEEM - HR LS CC/3(PwrXDecel), TEEM - HS LC CR/3(PwrXDecel)
  [K_PXeffSR] -> Multiport Switch1/6
  [K_PXeffRS] -> Multiport Switch1/7
  [K_PXeffCS] -> Multiport Switch1/5
  [K_PXeffSC] -> Multiport Switch1/4
  [K_PXeffRC] -> Multiport Switch1/2
  [K_PXeffCR] -> Multiport Switch1/3
  Constant3/1 -> Multiport Switch1/1
  Multiport Switch1/1 -> [K_PXeffL]
  [K_PXeffL] -> TEEM - HS LR CC/5(K_PXeffL), TEEM - HC LR CS/5(K_PXeffL), TEEM - HC LS CR/5(K_PXeffL), TEEM - HR LC CS/5(K_PXeffL), TEEM - HR LS CC/5(K_PXeffL), TEEM - HS LC CR/5(K_PXeffL)
  [PwrExAccel_TEEM] -> TEEM - HS LR CC/2(PwrExAccel), TEEM - HC LR CS/2(PwrExAccel), TEEM - HC LS CR/2(PwrExAccel), TEEM - HR LC CS/2(PwrExAccel), TEEM - HR LS CC/2(PwrExAccel), TEEM - HS LC CR/2(PwrExAccel)

== system AGTF30SysDyn_PExPIn/Control System/Scheduling/Steady State EM Power - MaxMin/HP and LP Pwr Calc/Gearbox Speeds/Spool to PGB speeds/Epicyclic Gearbox Speed Calc - RC ==
  NR : Inport
  NC : Inport  Port=2
  Gain1 : Gain  Gain=rP_I
  Gain2 : Gain  Gain=rS_M
  Gain30 : Gain  Gain=rR_M/rP_I
  Gain31 : Gain  Gain=1/rS_M
  Mux4 : Mux
  Sum : Sum  Inputs=|+-
  Sum2 : Sum  Inputs=|+-
  N : Outport
  wires:
  NC/1 -> Gain2/1, Mux4/3, Sum/2  "NC"
  NR/1 -> Mux4/2, Sum/1  "NR"
  Mux4/1 -> N/1
  Sum/1 -> Gain30/1
  Gain30/1 -> Mux4/4, Gain1/1  "NP"
  Gain1/1 -> Sum2/2
  Gain2/1 -> Sum2/1
  Sum2/1 -> Gain31/1
  Gain31/1 -> Mux4/1  "NS"

== system AGTF30SysDyn_PExPIn/Control System/Scheduling/Steady State EM Power - MaxMin/HP and LP Pwr Calc/Gearbox Speeds/Spool to PGB speeds/Epicyclic Gearbox Speed Calc - RC1 ==
  NR : Inport
  NC : Inport  Port=2
  Gain1 : Gain  Gain=rP_I
  Gain2 : Gain  Gain=rS_M
  Gain30 : Gain  Gain=rR_M/rP_I
  Gain31 : Gain  Gain=1/rS_M
  Mux4 : Mux
  Sum : Sum  Inputs=|+-
  Sum2 : Sum  Inputs=|+-
  N : Outport
  wires:
  Gain31/1 -> Mux4/1  "NS"
  Sum2/1 -> Gain31/1
  Gain2/1 -> Sum2/1
  Gain1/1 -> Sum2/2
  Gain30/1 -> Gain1/1, Mux4/4  "NP"
  Sum/1 -> Gain30/1
  Mux4/1 -> N/1
  NR/1 -> Sum/1, Mux4/2  "NR"
  NC/1 -> Sum/2, Mux4/3, Gain2/1  "NC"

== system AGTF30SysDyn_PExPIn/Control System/Scheduling/Steady State EM Power - MaxMin/HP and LP Pwr Calc/Gearbox Speeds/Spool to PGB speeds/Epicyclic Gearbox Speed Calc - SC ==
  NS : Inport
  NC : Inport  Port=2
  Gain1 : Gain  Gain=rP_I
  Gain2 : Gain  Gain=rR_M
  Gain30 : Gain  Gain=rS_M/rP_I
  Gain31 : Gain  Gain=1/rR_M
  Mux4 : Mux
  Sum : Sum  Inputs=|-+
  Sum1 : Sum  Inputs=|++
  N : Outport
  wires:
  Mux4/1 -> N/1
  Gain31/1 -> Mux4/2  "NR"
  Gain30/1 -> Mux4/4, Gain1/1  "NP"
  NS/1 -> Sum/1, Mux4/1  "NS"
  Sum1/1 -> Gain31/1
  NC/1 -> Gain2/1, Mux4/3, Sum/2  "NC"
  Sum/1 -> Gain30/1
  Gain1/1 -> Sum1/1
  Gain2/1 -> Sum1/2

== system AGTF30SysDyn_PExPIn/Control System/Scheduling/Steady State EM Power - MaxMin/HP and LP Pwr Calc/Gearbox Speeds/Spool to PGB speeds/Epicyclic Gearbox Speed Calc - SC1 ==
  NS : Inport
  NC : Inport  Port=2
  Gain1 : Gain  Gain=rP_I
  Gain2 : Gain  Gain=rR_M
  Gain30 : Gain  Gain=rS_M/rP_I
  Gain31 : Gain  Gain=1/rR_M
  Mux4 : Mux
  Sum : Sum  Inputs=|-+
  Sum1 : Sum  Inputs=|++
  N : Outport
  wires:
  Gain2/1 -> Sum1/2
  Gain1/1 -> Sum1/1
  Sum/1 -> Gain30/1
  NC/1 -> Sum/2, Mux4/3, Gain2/1  "NC"
  Sum1/1 -> Gain31/1
  NS/1 -> Mux4/1, Sum/1  "NS"
  Gain30/1 -> Gain1/1, Mux4/4  "NP"
  Gain31/1 -> Mux4/2  "NR"
  Mux4/1 -> N/1

== system AGTF30SysDyn_PExPIn/Control System/Scheduling/Steady State EM Power - MaxMin/HP and LP Pwr Calc/Gearbox Speeds/Spool to PGB speeds/Epicyclic Gearbox Speed Calc - SR ==
  NS : Inport
  NR : Inport  Port=2
  Gain : Gain  Gain=rS_M
  Gain29 : Gain  Gain=rR_M
  Gain30 : Gain  Gain=1/(rS_M+rR_M)
  Gain31 : Gain  Gain=rS_M/rP_I
  Mux4 : Mux
  Sum : Sum  Inputs=|++
  Sum1 : Sum  Inputs=-+|
  N : Outport
  wires:
  NS/1 -> Mux4/1, Mux4/3, Sum1/1, Gain/1
  Sum/1 -> Gain30/1
  Gain29/1 -> Sum/2
  NR/1 -> Mux4/2, Gain29/1
  Sum1/1 -> Gain31/1
  Gain/1 -> Sum/1
  Gain30/1 -> Sum1/2  "NC"
  Gain31/1 -> Mux4/4  "NP"
  Mux4/1 -> N/1

== system AGTF30SysDyn_PExPIn/Control System/Scheduling/Steady State EM Power - MaxMin/HP and LP Pwr Calc/Gearbox Speeds/Spool to PGB speeds/Epicyclic Gearbox Speed Calc - SR1 ==
  NS : Inport
  NR : Inport  Port=2
  Gain : Gain  Gain=rS_M
  Gain29 : Gain  Gain=rR_M
  Gain30 : Gain  Gain=1/(rS_M+rR_M)
  Gain31 : Gain  Gain=rS_M/rP_I
  Mux4 : Mux
  Sum : Sum  Inputs=|++
  Sum1 : Sum  Inputs=-+|
  N : Outport
  wires:
  Mux4/1 -> N/1
  Gain31/1 -> Mux4/4  "NP"
  Gain30/1 -> Sum1/2  "NC"
  Gain/1 -> Sum/1
  Sum1/1 -> Gain31/1
  NR/1 -> Gain29/1, Mux4/2
  Gain29/1 -> Sum/2
  Sum/1 -> Gain30/1
  NS/1 -> Gain/1, Sum1/1, Mux4/3, Mux4/1

== system AGTF30SysDyn_PExPIn/EngineSystem/Power System/Electrical Power System/EM Variant Subsystem/Scalar DEM Subsystem/PCabqPEM Calc/Zero Check2 ==
  EMPwr : Inport
  Abs : Abs  SaturateOnIntegerOverflow=off
  Compare To Constant : simulink/Logic and Bit Operations/Compare To Constant  relop=<=  const=1e-20  OutDataTypeStr=boolean
  Compare To Zero : simulink/Logic and Bit Operations/Compare To Zero  relop===  OutDataTypeStr=boolean
  Constant : Constant  Value=1e-20
  Divide : Product  Inputs=**
  Sign : Signum
  Switch : Switch  Criteria=u2 > Threshold  SaturateOnIntegerOverflow=off  InputSameDT=off
  Switch1 : Switch  Criteria=u2 > Threshold  SaturateOnIntegerOverflow=off  InputSameDT=off
  EMPwrNZ : Outport
  Check : Outport  Port=2
  wires:
  EMPwr/1 -> Compare To Zero/1, Sign/1, Switch/3, Abs/1
  Abs/1 -> Compare To Constant/1
  Compare To Zero/1 -> Switch1/2
  Sign/1 -> Divide/1
  Constant/1 -> Switch1/1, Divide/2
  Divide/1 -> Switch/1
  Switch/1 -> Switch1/3
  Compare To Constant/1 -> Check/1, Switch/2
  Switch1/1 -> EMPwrNZ/1

== system AGTF30SysDyn_PExPIn/EngineSystem/Power System/Electrical Power System/EM Variant Subsystem/Scalar DEM Subsystem/PCabqPEM Calc1/Zero Check2 ==
  EMPwr : Inport
  Abs : Abs  SaturateOnIntegerOverflow=off
  Compare To Constant : simulink/Logic and Bit Operations/Compare To Constant  relop=<=  const=1e-20  OutDataTypeStr=boolean
  Compare To Zero : simulink/Logic and Bit Operations/Compare To Zero  relop===  OutDataTypeStr=boolean
  Constant : Constant  Value=1e-20
  Divide : Product  Inputs=**
  Sign : Signum
  Switch : Switch  Criteria=u2 > Threshold  SaturateOnIntegerOverflow=off  InputSameDT=off
  Switch1 : Switch  Criteria=u2 > Threshold  SaturateOnIntegerOverflow=off  InputSameDT=off
  EMPwrNZ : Outport
  Check : Outport  Port=2
  wires:
  Switch1/1 -> EMPwrNZ/1
  Compare To Constant/1 -> Switch/2, Check/1
  Switch/1 -> Switch1/3
  Divide/1 -> Switch/1
  Constant/1 -> Divide/2, Switch1/1
  Sign/1 -> Divide/1
  Compare To Zero/1 -> Switch1/2
  Abs/1 -> Compare To Constant/1
  EMPwr/1 -> Abs/1, Switch/3, Sign/1, Compare To Zero/1

== system AGTF30SysDyn_PExPIn/EngineSystem/Power System/Electrical Power System/EM Variant Subsystem/Scalar PGB EM Subsystem/PCabqPEM Calc/Zero Check2 ==
  EMPwr : Inport
  Abs : Abs  SaturateOnIntegerOverflow=off
  Compare To Constant : simulink/Logic and Bit Operations/Compare To Constant  relop=<=  const=1e-20  OutDataTypeStr=boolean
  Compare To Zero : simulink/Logic and Bit Operations/Compare To Zero  relop===  OutDataTypeStr=boolean
  Constant : Constant  Value=1e-20
  Divide : Product  Inputs=**
  Sign : Signum
  Switch : Switch  Criteria=u2 > Threshold  SaturateOnIntegerOverflow=off  InputSameDT=off
  Switch1 : Switch  Criteria=u2 > Threshold  SaturateOnIntegerOverflow=off  InputSameDT=off
  EMPwrNZ : Outport
  Check : Outport  Port=2
  wires:
  EMPwr/1 -> Compare To Zero/1, Sign/1, Switch/3, Abs/1
  Abs/1 -> Compare To Constant/1
  Compare To Zero/1 -> Switch1/2
  Sign/1 -> Divide/1
  Constant/1 -> Switch1/1, Divide/2
  Divide/1 -> Switch/1
  Switch/1 -> Switch1/3
  Compare To Constant/1 -> Check/1, Switch/2
  Switch1/1 -> EMPwrNZ/1

== system AGTF30SysDyn_PExPIn/EngineSystem/Power System/Electrical Power System/EM Variant Subsystem/Scalar PGB EM Subsystem/PCabqPEM Calc1/Zero Check2 ==
  EMPwr : Inport
  Abs : Abs  SaturateOnIntegerOverflow=off
  Compare To Constant : simulink/Logic and Bit Operations/Compare To Constant  relop=<=  const=1e-20  OutDataTypeStr=boolean
  Compare To Zero : simulink/Logic and Bit Operations/Compare To Zero  relop===  OutDataTypeStr=boolean
  Constant : Constant  Value=1e-20
  Divide : Product  Inputs=**
  Sign : Signum
  Switch : Switch  Criteria=u2 > Threshold  SaturateOnIntegerOverflow=off  InputSameDT=off
  Switch1 : Switch  Criteria=u2 > Threshold  SaturateOnIntegerOverflow=off  InputSameDT=off
  EMPwrNZ : Outport
  Check : Outport  Port=2
  wires:
  EMPwr/1 -> Compare To Zero/1, Sign/1, Switch/3, Abs/1
  Abs/1 -> Compare To Constant/1
  Compare To Zero/1 -> Switch1/2
  Sign/1 -> Divide/1
  Constant/1 -> Switch1/1, Divide/2
  Divide/1 -> Switch/1
  Switch/1 -> Switch1/3
  Compare To Constant/1 -> Check/1, Switch/2
  Switch1/1 -> EMPwrNZ/1

== system AGTF30SysDyn_PExPIn/EngineSystem/Power System/Electrical Power System/EM Variant Subsystem/Scalar PGB EM Subsystem/PCabqPEM Calc2/Zero Check2 ==
  EMPwr : Inport
  Abs : Abs  SaturateOnIntegerOverflow=off
  Compare To Constant : simulink/Logic and Bit Operations/Compare To Constant  relop=<=  const=1e-20  OutDataTypeStr=boolean
  Compare To Zero : simulink/Logic and Bit Operations/Compare To Zero  relop===  OutDataTypeStr=boolean
  Constant : Constant  Value=1e-20
  Divide : Product  Inputs=**
  Sign : Signum
  Switch : Switch  Criteria=u2 > Threshold  SaturateOnIntegerOverflow=off  InputSameDT=off
  Switch1 : Switch  Criteria=u2 > Threshold  SaturateOnIntegerOverflow=off  InputSameDT=off
  EMPwrNZ : Outport
  Check : Outport  Port=2
  wires:
  EMPwr/1 -> Compare To Zero/1, Sign/1, Switch/3, Abs/1
  Abs/1 -> Compare To Constant/1
  Compare To Zero/1 -> Switch1/2
  Sign/1 -> Divide/1
  Constant/1 -> Switch1/1, Divide/2
  Divide/1 -> Switch/1
  Switch/1 -> Switch1/3
  Compare To Constant/1 -> Check/1, Switch/2
  Switch1/1 -> EMPwrNZ/1

== system AGTF30SysDyn_PExPIn/EngineSystem/Power System/Electrical Power System/EM Variant Subsystem/Scalar PGB EM Subsystem/PCabqPEM Calc3/Zero Check2 ==
  EMPwr : Inport
  Abs : Abs  SaturateOnIntegerOverflow=off
  Compare To Constant : simulink/Logic and Bit Operations/Compare To Constant  relop=<=  const=1e-20  OutDataTypeStr=boolean
  Compare To Zero : simulink/Logic and Bit Operations/Compare To Zero  relop===  OutDataTypeStr=boolean
  Constant : Constant  Value=1e-20
  Divide : Product  Inputs=**
  Sign : Signum
  Switch : Switch  Criteria=u2 > Threshold  SaturateOnIntegerOverflow=off  InputSameDT=off
  Switch1 : Switch  Criteria=u2 > Threshold  SaturateOnIntegerOverflow=off  InputSameDT=off
  EMPwrNZ : Outport
  Check : Outport  Port=2
  wires:
  EMPwr/1 -> Compare To Zero/1, Sign/1, Switch/3, Abs/1
  Abs/1 -> Compare To Constant/1
  Compare To Zero/1 -> Switch1/2
  Sign/1 -> Divide/1
  Constant/1 -> Switch1/1, Divide/2
  Divide/1 -> Switch/1
  Switch/1 -> Switch1/3
  Compare To Constant/1 -> Check/1, Switch/2
  Switch1/1 -> EMPwrNZ/1
